simulink model "sampleModel1503_4_sub_sub"  (R2023a)
settings: Solver=VariableStepAuto  StartTime=0.0  StopTime=10.0  RelTol=1e-3
libraries: hdlsllib x4
settings Model: Creator=user1  LastModifiedBy=user1

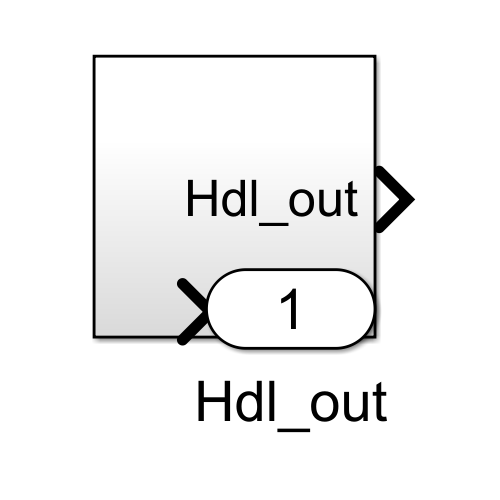
[thumbnail: Simulink's stored preview of the top-level diagram]
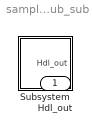
== system sampleModel1503_4_sub_sub ==
  Subsystem : Subsystem
  Hdl_out : Outport  OutDataTypeStr=uint8

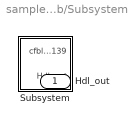
== system sampleModel1503_4_sub_sub/Subsystem ==
  Subsystem : Subsystem
  Hdl_out : Outport  OutDataTypeStr=uint8

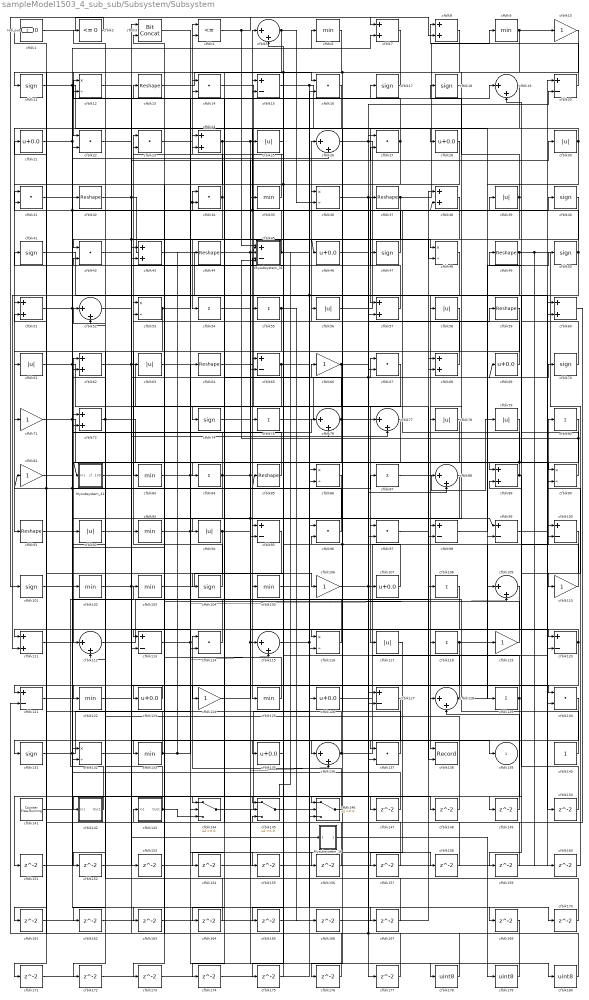
== system sampleModel1503_4_sub_sub/Subsystem/Subsystem ==
  Mysubsystem_16 : Subsystem  TreatAsAtomicUnit=on  RTWFcnName=Mysubsystem_16
      settings: RTWFcnNameOpts=User specified  RTWFileNameOpts=Use function name
  Mysubsystem_31 : Subsystem  TreatAsAtomicUnit=on  RTWFcnName=Mysubsystem_31
      settings: RTWFcnNameOpts=User specified  RTWFileNameOpts=Use function name
  Mysubsystem_41 : Subsystem  TreatAsAtomicUnit=on  RTWFcnName=Mysubsystem_41
      settings: RTWFcnNameOpts=User specified  RTWFileNameOpts=Use function name
  cfblk1 : hdlsllib/Logic and Bit Operations/Compare To Zero  relop=<=  OutDataTypeStr=uint8
  cfblk{10,66,71,81,106,110,119,124} (8 alike) : Gain  OutDataTypeStr=uint8
  cfblk{15,20,45,65,95,98..100,113,120..121,127} (12 alike) : Sum  Inputs=+-  OutDataTypeStr=uint8
  cfblk{11,17..18,40..41,47,50,70,74,101,104,131} (12 alike) : Signum
  cfblk{6,9,35,83,93,102..103,105,122,125,133} (11 alike) : MinMax  OutDataTypeStr=uint8
  cfblk{21,28,46,69,107,123,126,135} (8 alike) : Bias  Bias=0.0  SaturateOnIntegerOverflow=off
  cfblk{54..55,75,80,84,87,108,118,129} (9 alike) : Sum  Inputs=+  OutDataTypeStr=uint8
  cfblk{5,19,26,52,76..77,88,109,112,115,128,136} (12 alike) : Sum  Inputs=|++  OutDataTypeStr=uint8
  cfblk{7..8,24,38,43,51,57,60,62,68,72,89,111} (13 alike) : Sum  OutDataTypeStr=uint8
  cfblk{14,16,22..23,27,31,34,42,67,96..97,114,130,137} (14 alike) : DotProduct  OutDataTypeStr=uint8
  cfblk{12,36,48,53,86,90,116,132} (8 alike) : Product  Inputs=*/  OutDataTypeStr=uint8  RndMeth=Zero  SaturateOnIntegerOverflow=on
  cfblk{25,30,39,56,58,61,63,78..79,92,94,117} (12 alike) : Abs  OutDataTypeStr=uint8  SaturateOnIntegerOverflow=off
  cfblk{13,32,37,44,49,59,64,85,91} (9 alike) : Reshape
  cfblk138 : Record  FileSettingsInternal="{\"entries\":[{\"content\":{\"excelSettings\":{\"content\":{},\"type\":\"Streamout.ExcelSettings\"}},\"type\":\"Streamout.FileSettingStorage\",\"uuid\":\"\"}],\"packageUris\":[\"http:\\/\\/schema.mathworks.com\\/mf0\\/streamout_blocks\\/R2020a\"],\"version\":\"1.0\"}"  Layout=[1 1]  SignalsInternal="{\"entries\":[{\"content\":{\"signals\":[{\"content\":{\"blockPath\":[],\"dimensions\":[1],\"domain\":\"\",\"lineColor\":\"#a2142f\",\"plots\":[1],\"port\":1,\"signalID\":22240,\"signalName\":\"cfblk26\"},\"type\":\"RecordBlkView.Signal\",\"uuid\":\"\"},{\"content\":{\"blockPath\":[],\"dimensions\":[1],\"domain\":\"\",\"lineColor\":\"#139fff\",\"plots\":[1],\"port\":2,\"signalID\":22243,\"signalName\":\"cfblk97\"},\"type\":\"RecordBlkView.Signal\",\"uuid\":\"\"}]},\"type\":\"RecordBlkView.InputSignals\",\"uuid\":\"\"}],\"packageUris\":[\"http:\\/\\/schema.mathworks.com\\/mf0\\/streamout_blocks\\/R2020a\"],\"version\":\"1.0\"}"  VisualizationBindings="{\"xyplotplugin\":{\"info\":[{\"series\":[{\"bindingParametersList\":[{\"parameter\":\"X-Axis\",\"signalID\":22240,\"signalName\":\"cfblk26\"},{\"parameter\":\"Y-Axis\",\"signalID\":22243,\"signalName\":\"cfblk97\"}],\"seriesID\":12253}],\"subplotID\":1}]}}"  CompatibilityTag=XY  st=-1
  cfblk140 : Constant  OutDataTypeStr=uint8  SampleTime=-1
  cfblk141 : hdlsllib/Sources/Counter Free-Running  NumBits=16  tsamp=-1
  cfblk142 : Subsystem
      settings: LibrarySourceBlock=|
      | hdlsllib/Ports &
      | Subsystems/Subsystem
  cfblk143 : Subsystem
      settings: LibrarySourceBlock=|
      | hdlsllib/Ports &
      | Subsystems/Subsystem
  cfblk144 : Switch  OutDataTypeStr=uint8  SaturateOnIntegerOverflow=off  InputSameDT=off
  cfblk145 : Switch  OutDataTypeStr=uint8  SaturateOnIntegerOverflow=off  InputSameDT=off
  cfblk146 : Switch  OutDataTypeStr=uint8  SaturateOnIntegerOverflow=off  InputSameDT=off
  cfblk{147..167,169..177} (30 alike) : Delay  SampleTime=1
  cfblk178 : DataTypeConversion  OutDataTypeStr=uint8  SaturateOnIntegerOverflow=off  RndMeth=Floor
  cfblk179 : DataTypeConversion  OutDataTypeStr=uint8  SaturateOnIntegerOverflow=off  RndMeth=Floor
  cfblk180 : DataTypeConversion  OutDataTypeStr=uint8  SaturateOnIntegerOverflow=off  RndMeth=Floor
  cfblk2 : hdlsllib/Logic and Bit Operations/Compare To Zero  relop=<=  OutDataTypeStr=uint8
  cfblk3 : hdlsllib/Logic and Bit Operations/Bit Concat  numInputs=2
  cfblk4 : RelationalOperator  Operator=<=  OutDataTypeStr=boolean  InputSameDT=off
  cfblk139 : Outport  OutDataTypeStr=uint8  VectorParamsAs1DForOutWhenUnconnected=off
  Hdl_out : Outport  Port=2  OutDataTypeStr=uint8
  wires:
  Mysubsystem_41/1(cfblk139) -> cfblk139/1
  Mysubsystem_31/1(Out1) -> cfblk147/1
  Mysubsystem_16/1(Out1) -> cfblk179/1
  cfblk180/1 -> cfblk3/2
  cfblk179/1 -> cfblk3/1
  cfblk178/1 -> cfblk27/1, cfblk5/2
  cfblk177/1 -> cfblk1/1
  cfblk106/1 -> cfblk177/1
  cfblk176/1 -> cfblk53/2
  cfblk175/1 -> cfblk15/2
  cfblk174/1 -> cfblk116/2
  cfblk173/1 -> cfblk146/2
  cfblk172/1 -> cfblk146/3
  cfblk171/1 -> cfblk76/2
  cfblk170/1 -> cfblk145/3
  cfblk169/1 -> cfblk121/2
  cfblk167/1 -> cfblk43/1
  cfblk166/1 -> cfblk38/1
  cfblk165/1 -> cfblk68/2
  cfblk164/1 -> cfblk112/2
  cfblk163/1 -> cfblk127/2
  cfblk162/1 -> cfblk67/2
  cfblk108/1 -> cfblk162/1
  cfblk161/1 -> cfblk57/2
  cfblk160/1 -> cfblk90/2
  cfblk159/1 -> cfblk51/2
  cfblk158/1 -> cfblk24/2
  cfblk157/1 -> cfblk62/2
  cfblk117/1 -> cfblk157/1
  cfblk156/1 -> cfblk96/1
  cfblk155/1 -> cfblk60/2
  cfblk63/1 -> cfblk155/1
  cfblk154/1 -> cfblk137/2
  cfblk153/1 -> cfblk145/2
  cfblk42/1 -> cfblk153/1
  cfblk152/1 -> cfblk86/2
  cfblk95/1 -> cfblk152/1
  cfblk151/1 -> cfblk22/2
  cfblk150/1 -> cfblk19/2
  cfblk99/1 -> cfblk150/1
  cfblk149/1 -> cfblk128/2
  cfblk100/1 -> cfblk149/1
  cfblk148/1 -> cfblk52/2
  cfblk147/1 -> cfblk132/1
  cfblk31/1 -> cfblk97/2
  cfblk105/1 -> cfblk120/1
  cfblk141/1 -> cfblk26/2
  cfblk71/1 -> cfblk97/1, cfblk148/1
  cfblk5/1 -> cfblk61/1, cfblk36/2
  cfblk75/1 -> cfblk20/1
  cfblk22/1 -> cfblk137/1
  cfblk94/1 -> cfblk171/1, cfblk180/1
  cfblk115/1 -> cfblk70/1, cfblk130/2
  cfblk54/1 -> cfblk115/1, cfblk158/1
  cfblk70/1 -> cfblk39/1
  cfblk27/1 -> cfblk164/1, cfblk165/1, cfblk2/1
  cfblk102/1 -> cfblk114/2, cfblk7/2
  cfblk127/1 -> cfblk132/2
  cfblk112/1 -> cfblk68/1
  cfblk122/1 -> cfblk128/1
  cfblk143/1(Out1) -> cfblk144/3, cfblk92/1
  cfblk28/1 -> cfblk133/1
  cfblk57/1 -> cfblk37/1
  cfblk67/1 -> cfblk84/1
  cfblk145/1 -> cfblk126/1
  cfblk19/1 -> cfblk146/1
  cfblk130/1 -> cfblk131/1
  cfblk72/1 -> cfblk95/2, cfblk42/2
  cfblk61/1 -> cfblk108/1, cfblk163/1
  cfblk51/1 -> cfblk40/1, cfblk90/1
  cfblk77/1 -> cfblk144/2
  cfblk96/1 -> cfblk81/1, cfblk31/1
  cfblk21/1 -> cfblk112/1, cfblk6/1
  cfblk20/1 -> cfblk8/1
  cfblk81/1 -> cfblk19/1
  cfblk88/1 -> cfblk124/1
  cfblk83/1 -> cfblk88/1, cfblk156/1
  cfblk123/1 -> cfblk121/1
  cfblk65/1 -> cfblk98/2, cfblk113/2
  cfblk7/1 -> cfblk145/1, cfblk136/1
  cfblk32/1 -> cfblk77/2
  cfblk113/1 -> cfblk109/2, cfblk135/1
  cfblk23/1 -> cfblk4/2
  cfblk86/1 -> cfblk95/1
  cfblk110/1 -> cfblk89/2
  cfblk12/1 -> Mysubsystem_16/1(In1), cfblk46/1
  cfblk101/1 -> cfblk38/2, cfblk17/1
  cfblk137/1 -> cfblk36/1
  cfblk11/1 -> cfblk109/1, cfblk170/1
  cfblk92/1 -> cfblk67/1
  cfblk55/1 -> cfblk65/2, cfblk166/1
  cfblk120/1 -> cfblk111/1, cfblk154/1
  cfblk3/1 -> cfblk178/1
  cfblk109/1 -> cfblk144/1
  cfblk52/1 -> cfblk43/2
  cfblk144/1 -> cfblk16/2
  cfblk76/1 -> cfblk69/1, cfblk59/1, cfblk24/1, cfblk113/1
  cfblk133/1 -> cfblk87/1, cfblk44/1, cfblk21/1
  cfblk118/1 -> cfblk119/1, cfblk172/1
  cfblk84/1 -> cfblk118/1, cfblk27/2, cfblk12/2, cfblk173/1
  cfblk39/1 -> cfblk98/1, cfblk18/1
  cfblk107/1 -> cfblk56/1, cfblk25/1
  cfblk128/1 -> cfblk100/1, cfblk96/2
  cfblk124/1 -> cfblk35/1
  cfblk60/1 -> cfblk143/1(In1)
  cfblk1/1 -> cfblk7/1
  cfblk43/1 -> cfblk127/1
  cfblk13/1 -> cfblk16/1
  cfblk125/1 -> cfblk23/2
  cfblk41/1 -> cfblk86/1, cfblk100/2
  cfblk132/1 -> Mysubsystem_31/2(In2), cfblk30/1
  cfblk17/1 -> cfblk11/1
  cfblk6/1 -> cfblk65/1
  cfblk36/1 -> cfblk129/1, cfblk120/2
  cfblk131/1 -> cfblk64/1, cfblk14/2
  cfblk140/1 -> cfblk102/1
  cfblk91/1 -> cfblk32/1
  cfblk90/1 -> cfblk49/1
  cfblk38/1 -> cfblk55/1
  cfblk85/1 -> cfblk63/1
  cfblk45/1 -> cfblk12/1, cfblk167/1
  cfblk97/1 -> cfblk138/2
  cfblk40/1 -> cfblk54/1
  cfblk129/1 -> cfblk41/1, cfblk151/1
  cfblk89/1 -> Mysubsystem_41/1(In1), cfblk31/2, cfblk159/1
  cfblk93/1 -> cfblk66/1, cfblk115/2
  cfblk9/1 -> cfblk174/1, cfblk175/1, cfblk10/1
  cfblk58/1 -> cfblk142/1(In1)
  cfblk66/1 -> cfblk123/1, cfblk88/2
  cfblk111/1 -> cfblk72/1
  cfblk116/1 -> cfblk52/1
  cfblk10/1 -> cfblk78/1
  cfblk135/1 -> cfblk45/2
  cfblk119/1 -> cfblk93/1
  cfblk14/1 -> cfblk77/1
  cfblk59/1 -> cfblk83/1
  cfblk79/1 -> cfblk104/1
  cfblk47/1 -> cfblk5/1, cfblk14/1
  cfblk34/1 -> cfblk4/1, cfblk42/1
  cfblk80/1 -> Mysubsystem_31/3(In3), cfblk116/1
  cfblk103/1 -> cfblk106/1
  cfblk98/1 -> cfblk50/1
  cfblk44/1 -> cfblk45/1, cfblk48/1, cfblk130/1
  cfblk136/1 -> cfblk60/1, cfblk72/2
  cfblk46/1 -> cfblk107/1, cfblk169/1
  cfblk26/1 -> cfblk138/1, cfblk20/2
  cfblk87/1 -> cfblk79/1
  cfblk146/1 -> cfblk114/1
  cfblk121/1 -> cfblk85/1, cfblk76/1
  cfblk53/1 -> cfblk71/1, cfblk15/1
  cfblk50/1 -> cfblk34/1, cfblk34/2, cfblk111/2
  cfblk48/1 -> cfblk94/1
  cfblk2/1 -> cfblk101/1
  cfblk62/1 -> cfblk74/1, cfblk47/1
  cfblk24/1 -> cfblk117/1, cfblk48/2, cfblk51/1
  cfblk49/1 -> cfblk110/1, cfblk160/1, cfblk161/1
  cfblk35/1 -> cfblk13/1
  cfblk8/1 -> cfblk22/1
  cfblk30/1 -> cfblk28/1, cfblk99/2
  cfblk25/1 -> cfblk105/1
  cfblk15/1 -> cfblk57/1, cfblk58/1
  cfblk126/1 -> cfblk80/1
  cfblk74/1 -> cfblk99/1, cfblk136/2
  cfblk16/1 -> cfblk75/1
  cfblk18/1 -> cfblk91/1
  cfblk68/1 -> cfblk53/1
  cfblk114/1 -> cfblk62/1
  cfblk64/1 -> cfblk125/1
  cfblk56/1 -> cfblk89/1
  cfblk69/1 -> cfblk26/1
  cfblk142/1(Out1) -> cfblk103/1
  cfblk4/1 -> cfblk8/2, Mysubsystem_31/1(In1)
  cfblk37/1 -> cfblk9/1, cfblk176/1
  cfblk78/1 -> cfblk122/1
  cfblk104/1 -> cfblk23/1

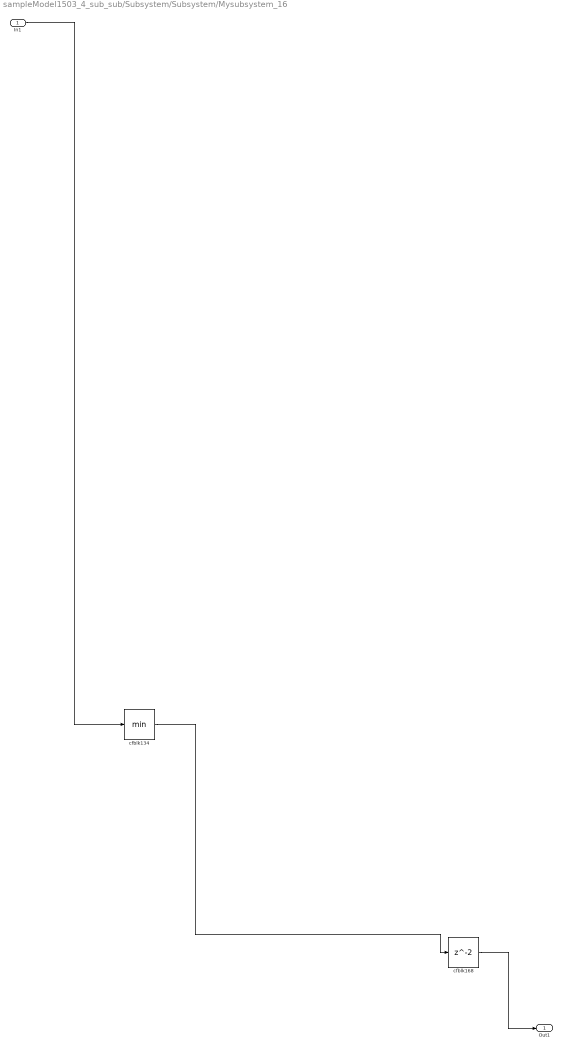
== system sampleModel1503_4_sub_sub/Subsystem/Subsystem/Mysubsystem_16 ==
  In1 : Inport
  cfblk134 : MinMax
  cfblk168 : Delay  SampleTime=1
  Out1 : Outport
  wires:
  cfblk134/1 -> cfblk168/1
  cfblk168/1 -> Out1/1
  In1/1 -> cfblk134/1

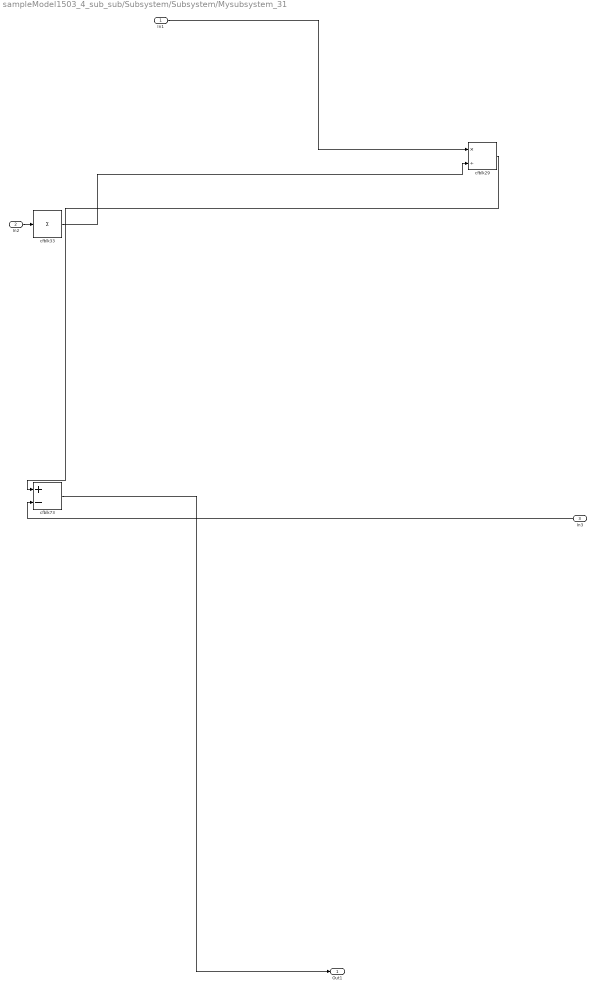
== system sampleModel1503_4_sub_sub/Subsystem/Subsystem/Mysubsystem_31 ==
  In1 : Inport
  In2 : Inport  Port=2
  In3 : Inport  Port=3
  cfblk29 : Product  Inputs=*/  RndMeth=Zero  SaturateOnIntegerOverflow=on
  cfblk33 : Sum  Inputs=+
  cfblk73 : Sum  Inputs=+-
  Out1 : Outport
  wires:
  In1/1 -> cfblk29/1
  cfblk29/1 -> cfblk73/1
  In2/1 -> cfblk33/1
  cfblk33/1 -> cfblk29/2
  cfblk73/1 -> Out1/1
  In3/1 -> cfblk73/2

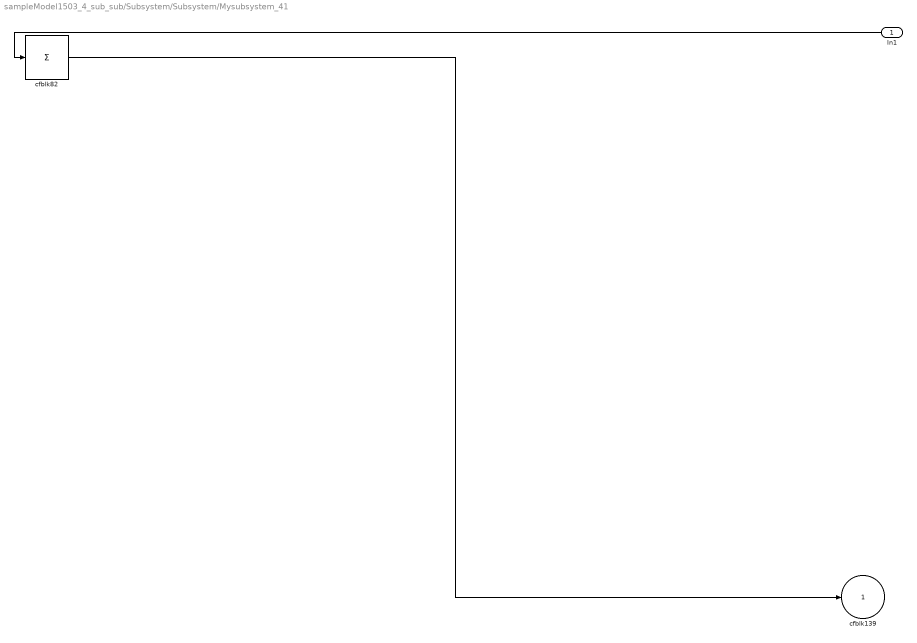
== system sampleModel1503_4_sub_sub/Subsystem/Subsystem/Mysubsystem_41 ==
  In1 : Inport
  cfblk82 : Sum  Inputs=+
  cfblk139 : Outport  VectorParamsAs1DForOutWhenUnconnected=off
  wires:
  cfblk82/1 -> cfblk139/1
  In1/1 -> cfblk82/1

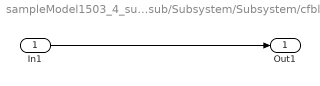
== system sampleModel1503_4_sub_sub/Subsystem/Subsystem/cfblk142 ==
  In1 : Inport
  Out1 : Outport
  wires:
  In1/1 -> Out1/1

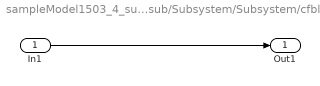
== system sampleModel1503_4_sub_sub/Subsystem/Subsystem/cfblk143 ==
  In1 : Inport
  Out1 : Outport
  wires:
  In1/1 -> Out1/1
